simulink model "stream_mdbrt_backup5"  (R2023b)
settings: Solver=VariableStepAuto  StartTime=0.0  StopTime=(48)/fs  RelTol=1e-3
PreLoadFcn:
  | clear all;
  | 
  | fs = 100e6;
PostLoadFcn:
  | ratio = 1/6;
  | set(0,'units','pixels');
  | pixels = get(0,'screensize');
  | point1 = round(pixels(3)*ratio);
  | point2 = round(pixels(4)*ratio);
  | point3 = pixels(3)-round(pixels(3)*ratio);
  | point4 = pixels(4)-round(pixels(4)*ratio);
  | h = get_param(gcs,'handle');
  | set_param(h,'location',[point1 point2 point3 point4]);
  | pause(0.2);
  | set_param(h,'Zoomfactor','fit to view');
  | 
  | clear ratio pixels point1 point2 point3 point4 h
  | 
  | % https://uk.mathworks.com/matlabcentral/answers/358413-open-simulink-model-with-set-window-size-and-position
undefined symbols (not defined in the file): AXI4, bits, bitsheight, bitsiter, bitswidth, Lite, xc7z020clg400
libraries: hdlBasic x527, vmcUtilities x1
(part 3 of 5)

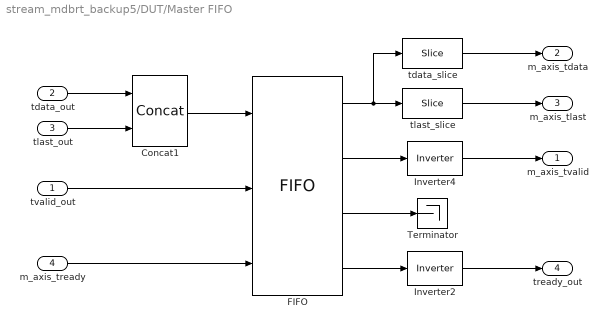
== system stream_mdbrt_backup5/DUT/Master FIFO ==
  tvalid_out : Inport
  tdata_out : Inport  Port=2
  tlast_out : Inport  Port=3
  m_axis_tready : Inport  Port=4
  Concat1 : hdlBasic/Concat  num_inputs=2  XmcBlockStatus=1  maskContainerNames=group1  block_type=concat  block_config=sysgen:Concat_config
  FIFO : hdlBasic/FIFO  mem_type=Block RAM  performance_options=First_Word_Fall_Through  embedded_registers=off  depth=1K  use_asym_data_widths=off  asym_read_width=32  percent_nbits=1  rst=off  rst_latency=1  en=off  use_dcount=off  use_percent_full_port=off  use_almost_empty=off  almost_empty_thresh=2  use_almost_full=on  use_rd_rst_busy=off  use_wr_rst_busy=off  almost_full_thresh=1000  almost_empty_offset=[]  almost_full_offset=[]  explicit_period=off  period=[]  store_only_valid=[]  init_zero=[]  simulation_type=fast_sim  XmcBlockStatus=1  maskContainerNames=tabcontainer1  block_type=fifo  block_config=sysgen:FIFO_config  block_width=538  block_height=997
      settings: infoedit=[]
  Inverter2 : hdlBasic/Inverter  en=off  latency=0  XmcBlockStatus=1  maskContainerNames=group2  block_type=inv  block_config=sysgen:Inverter_config
  Inverter4 : hdlBasic/Inverter  en=off  latency=0  XmcBlockStatus=1  maskContainerNames=group2  block_type=inv  block_config=sysgen:Inverter_config
  Terminator : Terminator
  tdata_slice : hdlBasic/Slice  nbits=1  boolean_output=off  mode=Two Bit Locations  bit1=0  base1=MSB of Input  bit0=1  base0=LSB of Input  XmcBlockStatus=1  maskContainerNames=group1  block_type=slice  block_config=sysgen:Slice_config
  tlast_slice : hdlBasic/Slice  nbits=1  boolean_output=on  mode=Two Bit Locations  bit1=0  base1=LSB of Input  bit0=0  base0=LSB of Input  XmcBlockStatus=1  maskContainerNames=group1  block_type=slice  block_config=sysgen:Slice_config
  m_axis_tvalid : Outport
  m_axis_tdata : Outport  Port=2
  m_axis_tlast : Outport  Port=3
  tready_out : Outport  Port=4
  wires:
  FIFO/4 -> Inverter2/1
  Inverter2/1 -> tready_out/1
  FIFO/2 -> Inverter4/1
  FIFO/1 -> tlast_slice/1, tdata_slice/1
  tlast_slice/1 -> m_axis_tlast/1
  tdata_slice/1 -> m_axis_tdata/1
  m_axis_tready/1 -> FIFO/3
  tvalid_out/1 -> FIFO/2
  Concat1/1 -> FIFO/1
  tdata_out/1 -> Concat1/1
  tlast_out/1 -> Concat1/2
  Inverter4/1 -> m_axis_tvalid/1
  FIFO/3 -> Terminator/1

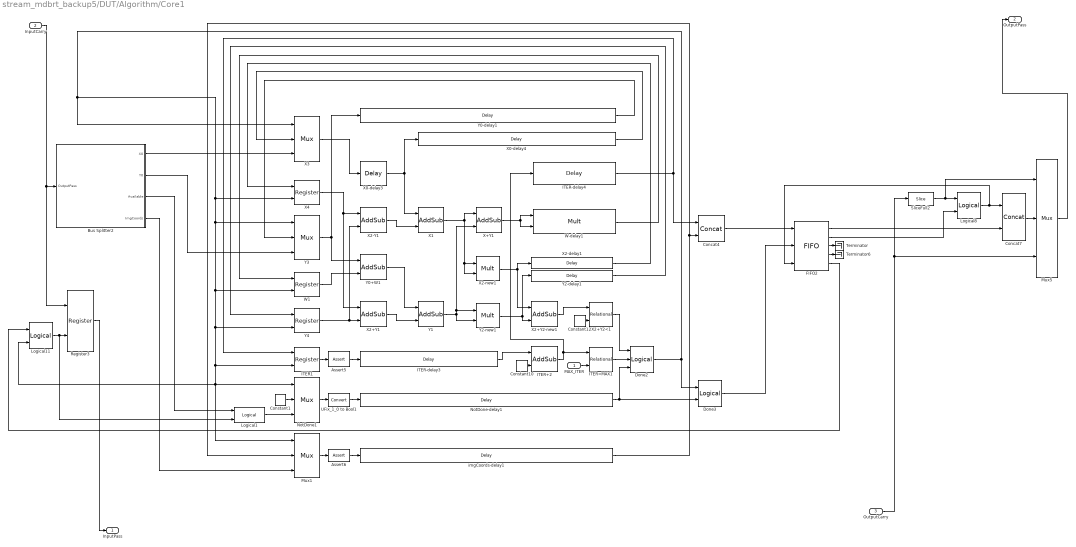
== system stream_mdbrt_backup5/DUT/Algorithm/Core1 ==
  MAX_ITER : Inport
  InputCarry : Inport  Port=2
  OutputCarry : Inport  Port=3
  Assert5 : hdlBasic/Assert  assert_type=on  type_source=Explicitly  gui_display_data_type=Fixed-point  arith_type=Unsigned  n_bits=bitsiter  bin_pt=0  preci_type=Single  exp_width=8  frac_width=24  assert_rate=off  rate_source=Explicitly  period=1  output_port=on  XmcBlockStatus=1  maskContainerNames=group1  block_type=assert  block_config=sysgen:assert_config  block_width=609  block_height=900
  Assert6 : hdlBasic/Assert  assert_type=on  type_source=Explicitly  gui_display_data_type=Fixed-point  arith_type=Unsigned  n_bits=bitswidth+bitsheight  bin_pt=0  preci_type=Single  exp_width=8  frac_width=24  assert_rate=off  rate_source=Explicitly  period=1  output_port=on  XmcBlockStatus=1  maskContainerNames=group1  block_type=assert  block_config=sysgen:assert_config  block_width=609  block_height=900
  Bus Splitter2 : Subsystem  TreatAsAtomicUnit=on
  Concat4 : hdlBasic/Concat  num_inputs=2  XmcBlockStatus=1  maskContainerNames=group1  block_type=concat  block_config=sysgen:Concat_config
  Concat7 : hdlBasic/Concat  num_inputs=2  XmcBlockStatus=1  maskContainerNames=group1  block_type=concat  block_config=sysgen:Concat_config
  Constant1 : hdlBasic/Constant  const=1  gui_display_data_type=Boolean  arith_type=Boolean  n_bits=bits  bin_pt=0  preci_type=Single  exp_width=8  frac_width=24  explicit_period=off  period=1  XmcBlockStatus=1  maskContainerNames=tabcontainer1  block_type=constant  block_config=sysgen:Constant_config
  Constant10 : hdlBasic/Constant  const=1  gui_display_data_type=Fixed-point  arith_type=Unsigned  n_bits=bits  bin_pt=0  preci_type=Single  exp_width=8  frac_width=24  explicit_period=off  period=1  XmcBlockStatus=1  maskContainerNames=tabcontainer1  block_type=constant  block_config=sysgen:Constant_config
  Constant12 : hdlBasic/Constant  const=4  gui_display_data_type=Fixed-point  arith_type=Signed (2's comp)  n_bits=bits  bin_pt=binpoint  preci_type=Single  exp_width=8  frac_width=24  explicit_period=off  period=1  XmcBlockStatus=1  maskContainerNames=tabcontainer1  block_type=constant  block_config=sysgen:Constant_config
  Done2 : hdlBasic/Logical  logical_function=NAND  inputs=3  en=off  latency=0  precision=User Defined  arith_type=Boolean  n_bits=1  bin_pt=0  align_bp=on  overflow=[]  quantization=[]  XmcBlockStatus=1  maskContainerNames=tabcontainer1  block_type=logical  block_config=sysgen:Logical_config
  Done3 : hdlBasic/Logical  logical_function=AND  inputs=2  en=off  latency=0  precision=User Defined  arith_type=Boolean  n_bits=1  bin_pt=0  align_bp=on  overflow=[]  quantization=[]  XmcBlockStatus=1  maskContainerNames=tabcontainer1  block_type=logical  block_config=sysgen:Logical_config
  FIFO2 : hdlBasic/FIFO  mem_type=Distributed RAM  performance_options=First_Word_Fall_Through  embedded_registers=off  depth=32  use_asym_data_widths=off  asym_read_width=32  percent_nbits=1  rst=off  rst_latency=1  en=off  use_dcount=off  use_percent_full_port=on  use_almost_empty=on  almost_empty_thresh=15  use_almost_full=off  use_rd_rst_busy=off  use_wr_rst_busy=off  almost_full_thresh=7  almost_empty_offset=[]  almost_full_offset=[]  explicit_period=off  period=[]  store_only_valid=[]  init_zero=[]  simulation_type=fast_sim  XmcBlockStatus=1  maskContainerNames=tabcontainer1  block_type=fifo  block_config=sysgen:FIFO_config  block_width=538  block_height=997
      settings: infoedit=[]
  ITER+2 : hdlBasic/AddSub  mode=Addition  use_carryin=off  use_carryout=off  en=off  latency=3  precision=User Defined  arith_type=Unsigned  n_bits=bitsiter  bin_pt=0  quantization=Truncate  overflow=Wrap  use_behavioral_HDL=off  hw_selection=Fabric  pipelined=off  XmcBlockStatus=1  maskContainerNames=tabcontainer1  block_type=addsub  block_config=sysgen:Addsub_config
  ITER-delay3 : hdlBasic/Delay  rst=off  en=off  latency=8  reg_retiming=off  XmcBlockStatus=1  maskContainerNames=group1  block_type=delay  block_config=sysgen:Delay_config
  ITER-delay4 : hdlBasic/Delay  rst=off  en=off  latency=2  reg_retiming=off  XmcBlockStatus=1  maskContainerNames=group1  block_type=delay  block_config=sysgen:Delay_config
  ITER1 : hdlBasic/Register  init=0  rst=on  en=off  XmcBlockStatus=1  maskContainerNames=tabcontainer1  block_type=register  block_config=sysgen:Register_config
  ITER<MAX1 : hdlBasic/Relational  mode=a<b  op_type=Bool  en=off  latency=2  XmcBlockStatus=1  maskContainerNames=tabcontainer1  block_type=relational  block_config=sysgen:Relational_config
  Logical1 : hdlBasic/Logical  logical_function=AND  inputs=2  en=off  latency=0  precision=Full  arith_type=Unsigned  n_bits=16  bin_pt=0  align_bp=on  overflow=[]  quantization=[]  XmcBlockStatus=1  maskContainerNames=tabcontainer1  block_type=logical  block_config=sysgen:Logical_config
  Logical11 : hdlBasic/Logical  logical_function=AND  inputs=2  en=off  latency=0  precision=Full  arith_type=Unsigned  n_bits=16  bin_pt=0  align_bp=on  overflow=[]  quantization=[]  XmcBlockStatus=1  maskContainerNames=tabcontainer1  block_type=logical  block_config=sysgen:Logical_config
  Logical8 : hdlBasic/Logical  logical_function=NOR  inputs=2  en=off  latency=0  precision=Full  arith_type=Unsigned  n_bits=16  bin_pt=0  align_bp=on  overflow=[]  quantization=[]  XmcBlockStatus=1  maskContainerNames=tabcontainer1  block_type=logical  block_config=sysgen:Logical_config
  Mux1 : hdlBasic/Mux  inputs=2  en=off  latency=1  precision=User Defined  arith_type=Unsigned  n_bits=bitswidth+bitsheight  bin_pt=0  quantization=Truncate  overflow=Wrap  XmcBlockStatus=1  maskContainerNames=tabcontainer1  block_type=mux  block_config=sysgen:Mux_config
  Mux5 : hdlBasic/Mux  inputs=2  en=off  latency=1  precision=User Defined  arith_type=Unsigned  n_bits=bitswidth+bitsheight+bitsiter+1  bin_pt=0  quantization=Truncate  overflow=Wrap  XmcBlockStatus=1  maskContainerNames=tabcontainer1  block_type=mux  block_config=sysgen:Mux_config
  NotDone-delay1 : hdlBasic/Delay  rst=off  en=off  latency=13  reg_retiming=off  XmcBlockStatus=1  maskContainerNames=group1  block_type=delay  block_config=sysgen:Delay_config
  NotDone1 : hdlBasic/Mux  inputs=2  en=off  latency=1  precision=User Defined  arith_type=Unsigned  n_bits=1  bin_pt=0  quantization=Truncate  overflow=Wrap  XmcBlockStatus=1  maskContainerNames=tabcontainer1  block_type=mux  block_config=sysgen:Mux_config
  Register3 : hdlBasic/Register  init=0  rst=on  en=off  XmcBlockStatus=1  maskContainerNames=tabcontainer1  block_type=register  block_config=sysgen:Register_config
  SliceFull2 : hdlBasic/Slice  nbits=1  boolean_output=on  mode=Upper Bit Location + Width  bit1=0  base1=MSB of Input  bit0=0  base0=LSB of Input  XmcBlockStatus=1  maskContainerNames=group1  block_type=slice  block_config=sysgen:Slice_config
  Terminator : Terminator
  Terminator6 : Terminator
  UFix_1_0 to Bool1 : hdlBasic/Convert  gui_display_data_type=Boolean  arith_type=Boolean  n_bits=16  bin_pt=14  float_type=Single  exp_bits=8  fraction_bits=24  quantization=Truncate  overflow=Wrap  en=off  latency=0  pipeline=off  XmcBlockStatus=1  maskContainerNames=group2  block_type=convert  block_config=sysgen:Convert_config  block_width=595  block_height=885
  W-delay1 : hdlBasic/Mult  precision=Full  arith_type="Signed  (2's comp)"  n_bits=16  bin_pt=14  quantization=Truncate  overflow=Wrap  en=off  latency=7  use_behavioral_HDL=off  opt=Speed  use_embedded=on  optimum_pipeline=off  pipeline=on  use_rpm=on  placement_style=Triangular  XmcBlockStatus=1  maskContainerNames=group1  block_type=mult  block_config=sysgen:Mult_config  block_width=598  block_height=876
  W1 : hdlBasic/Register  init=0  rst=on  en=off  XmcBlockStatus=1  maskContainerNames=tabcontainer1  block_type=register  block_config=sysgen:Register_config
  X+Y1 : hdlBasic/AddSub  mode=Addition  use_carryin=off  use_carryout=off  en=off  latency=4  precision=User Defined  arith_type="Signed  (2's comp)"  n_bits=bits  bin_pt=binpoint  quantization=Truncate  overflow=Wrap  use_behavioral_HDL=off  hw_selection=Fabric  pipelined=off  XmcBlockStatus=1  maskContainerNames=tabcontainer1  block_type=addsub  block_config=sysgen:Addsub_config
  X0-delay3 : hdlBasic/Delay  rst=off  en=off  latency=1  reg_retiming=off  XmcBlockStatus=1  maskContainerNames=group1  block_type=delay  block_config=sysgen:Delay_config
  X0-delay4 : hdlBasic/Delay  rst=off  en=off  latency=12  reg_retiming=off  XmcBlockStatus=1  maskContainerNames=group1  block_type=delay  block_config=sysgen:Delay_config
  X1 : hdlBasic/AddSub  mode=Addition  use_carryin=off  use_carryout=off  en=off  latency=1  precision=User Defined  arith_type="Signed  (2's comp)"  n_bits=bits  bin_pt=binpoint  quantization=Truncate  overflow=Wrap  use_behavioral_HDL=off  hw_selection=Fabric  pipelined=off  XmcBlockStatus=1  maskContainerNames=tabcontainer1  block_type=addsub  block_config=sysgen:Addsub_config
  X2+Y1 : hdlBasic/AddSub  mode=Addition  use_carryin=off  use_carryout=off  en=off  latency=1  precision=User Defined  arith_type="Signed  (2's comp)"  n_bits=bits  bin_pt=binpoint  quantization=Truncate  overflow=Wrap  use_behavioral_HDL=off  hw_selection=Fabric  pipelined=off  XmcBlockStatus=1  maskContainerNames=tabcontainer1  block_type=addsub  block_config=sysgen:Addsub_config
  X2+Y2-new1 : hdlBasic/AddSub  mode=Addition  use_carryin=off  use_carryout=off  en=off  latency=3  precision=User Defined  arith_type="Signed  (2's comp)"  n_bits=bits  bin_pt=binpoint  quantization=Truncate  overflow=Wrap  use_behavioral_HDL=off  hw_selection=Fabric  pipelined=off  XmcBlockStatus=1  maskContainerNames=tabcontainer1  block_type=addsub  block_config=sysgen:Addsub_config
  X2+Y2<1 : hdlBasic/Relational  mode=a<b  op_type=Bool  en=off  latency=2  XmcBlockStatus=1  maskContainerNames=tabcontainer1  block_type=relational  block_config=sysgen:Relational_config
  X2-Y1 : hdlBasic/AddSub  mode=Subtraction  use_carryin=off  use_carryout=off  en=off  latency=1  precision=User Defined  arith_type="Signed  (2's comp)"  n_bits=bits  bin_pt=binpoint  quantization=Truncate  overflow=Wrap  use_behavioral_HDL=off  hw_selection=Fabric  pipelined=off  XmcBlockStatus=1  maskContainerNames=tabcontainer1  block_type=addsub  block_config=sysgen:Addsub_config
  X2-delay1 : hdlBasic/Delay  rst=off  en=off  latency=5  reg_retiming=off  XmcBlockStatus=1  maskContainerNames=group1  block_type=delay  block_config=sysgen:Delay_config
  X2-new1 : hdlBasic/Mult  precision=Full  arith_type="Signed  (2's comp)"  n_bits=16  bin_pt=14  quantization=Truncate  overflow=Wrap  en=off  latency=6  use_behavioral_HDL=off  opt=Speed  use_embedded=on  optimum_pipeline=off  pipeline=on  use_rpm=on  placement_style=Triangular  XmcBlockStatus=1  maskContainerNames=group1  block_type=mult  block_config=sysgen:Mult_config  block_width=598  block_height=876
  X3 : hdlBasic/Mux  inputs=2  en=off  latency=1  precision=User Defined  arith_type="Signed  (2's comp)"  n_bits=bits  bin_pt=binpoint  quantization=Truncate  overflow=Wrap  XmcBlockStatus=1  maskContainerNames=tabcontainer1  block_type=mux  block_config=sysgen:Mux_config
  X4 : hdlBasic/Register  init=0  rst=on  en=off  XmcBlockStatus=1  maskContainerNames=tabcontainer1  block_type=register  block_config=sysgen:Register_config
  Y0+W1 : hdlBasic/AddSub  mode=Addition  use_carryin=off  use_carryout=off  en=off  latency=1  precision=User Defined  arith_type="Signed  (2's comp)"  n_bits=bits  bin_pt=binpoint  quantization=Truncate  overflow=Wrap  use_behavioral_HDL=off  hw_selection=Fabric  pipelined=off  XmcBlockStatus=1  maskContainerNames=tabcontainer1  block_type=addsub  block_config=sysgen:Addsub_config
  Y0-delay1 : hdlBasic/Delay  rst=off  en=off  latency=13  reg_retiming=off  XmcBlockStatus=1  maskContainerNames=group1  block_type=delay  block_config=sysgen:Delay_config
  Y1 : hdlBasic/AddSub  mode=Subtraction  use_carryin=off  use_carryout=off  en=off  latency=1  precision=User Defined  arith_type="Signed  (2's comp)"  n_bits=bits  bin_pt=binpoint  quantization=Truncate  overflow=Wrap  use_behavioral_HDL=off  hw_selection=Fabric  pipelined=off  XmcBlockStatus=1  maskContainerNames=tabcontainer1  block_type=addsub  block_config=sysgen:Addsub_config
  Y2-delay1 : hdlBasic/Delay  rst=off  en=off  latency=5  reg_retiming=off  XmcBlockStatus=1  maskContainerNames=group1  block_type=delay  block_config=sysgen:Delay_config
  Y2-new1 : hdlBasic/Mult  precision=Full  arith_type="Signed  (2's comp)"  n_bits=16  bin_pt=14  quantization=Truncate  overflow=Wrap  en=off  latency=6  use_behavioral_HDL=off  opt=Speed  use_embedded=on  optimum_pipeline=off  pipeline=on  use_rpm=on  placement_style=Triangular  XmcBlockStatus=1  maskContainerNames=group1  block_type=mult  block_config=sysgen:Mult_config  block_width=598  block_height=876
  Y3 : hdlBasic/Mux  inputs=2  en=off  latency=1  precision=User Defined  arith_type="Signed  (2's comp)"  n_bits=bits  bin_pt=binpoint  quantization=Truncate  overflow=Wrap  XmcBlockStatus=1  maskContainerNames=tabcontainer1  block_type=mux  block_config=sysgen:Mux_config
  Y4 : hdlBasic/Register  init=0  rst=on  en=off  XmcBlockStatus=1  maskContainerNames=tabcontainer1  block_type=register  block_config=sysgen:Register_config
  imgCoords-delay1 : hdlBasic/Delay  rst=off  en=off  latency=13  reg_retiming=off  XmcBlockStatus=1  maskContainerNames=group1  block_type=delay  block_config=sysgen:Delay_config
  InputPass : Outport
  OutputPass : Outport  Port=2
  wires:
  NotDone1/1 -> UFix_1_0 to Bool1/1
  SliceFull2/1 -> Mux5/1, Logical8/1
  ITER-delay3/1 -> ITER+2/1
  Y4/1 -> X2-Y1/2, X2+Y1/2
  Y2-delay1/1 -> Y4/1
  Done3/1 -> FIFO2/2
  Assert6/1 -> imgCoords-delay1/1
  InputCarry/1 -> Register3/1, Bus Splitter2/1(OutputPass)
  X1/1 -> X2-new1/2, X2-new1/1, X+Y1/1
  X2-delay1/1 -> X4/1
  Done2/1 -> Done3/1, X4/2, Y3/1, W1/2, ITER1/2, Logical11/2, Mux1/1, NotDone1/1, Y4/2, X3/1
  W1/1 -> Y0+W1/2
  Constant10/1 -> ITER+2/2
  Logical8/1 -> FIFO2/3, Concat7/1
  FIFO2/2 -> Logical8/2
  X2+Y2-new1/1 -> X2+Y2<1/1
  Bus Splitter2/1(X0) -> X3/3
  X2+Y1/1 -> Y1/2
  Logical11/1 -> Logical1/2, Register3/2
  NotDone-delay1/1 -> Done2/3, Done3/2
  OutputCarry/1 -> SliceFull2/1, Mux5/3
  Mux5/1 -> OutputPass/1
  FIFO2/3 -> Terminator/1
  ITER-delay4/1 -> Concat4/1, ITER1/1
  Y3/1 -> Y0+W1/1, Y0-delay1/1
  Register3/1 -> InputPass/1
  X4/1 -> X2+Y1/1, X2-Y1/1
  ITER+2/1 -> ITER-delay4/1, ITER<MAX1/1
  Y1/1 -> X+Y1/2, Y2-new1/1, Y2-new1/2
  Y2-new1/1 -> Y2-delay1/1, X2+Y2-new1/2
  ITER<MAX1/1 -> Done2/2
  Constant12/1 -> X2+Y2<1/2
  Y0+W1/1 -> Y1/1
  Assert5/1 -> ITER-delay3/1
  UFix_1_0 to Bool1/1 -> NotDone-delay1/1
  X2+Y2<1/1 -> Done2/1
  imgCoords-delay1/1 -> Mux1/2, Concat4/2
  FIFO2/5 -> Logical11/1
  Bus Splitter2/4(ImgCoords) -> Mux1/3
  X2-Y1/1 -> X1/2
  ITER1/1 -> Assert5/1
  X+Y1/1 -> W-delay1/2, W-delay1/1
  X0-delay3/1 -> X0-delay4/1, X1/1
  Y0-delay1/1 -> Y3/2
  X3/1 -> X0-delay3/1
  Concat7/1 -> Mux5/2
  X0-delay4/1 -> X3/2
  X2-new1/1 -> X2-delay1/1, X2+Y2-new1/1
  Bus Splitter2/2(Y0) -> Y3/3
  W-delay1/1 -> W1/1
  MAX_ITER/1 -> ITER<MAX1/2
  Bus Splitter2/3(Available) -> Logical1/1
  FIFO2/4 -> Terminator6/1
  Mux1/1 -> Assert6/1
  Concat4/1 -> FIFO2/1
  FIFO2/1 -> Concat7/2
  Constant1/1 -> NotDone1/2
  Logical1/1 -> NotDone1/3

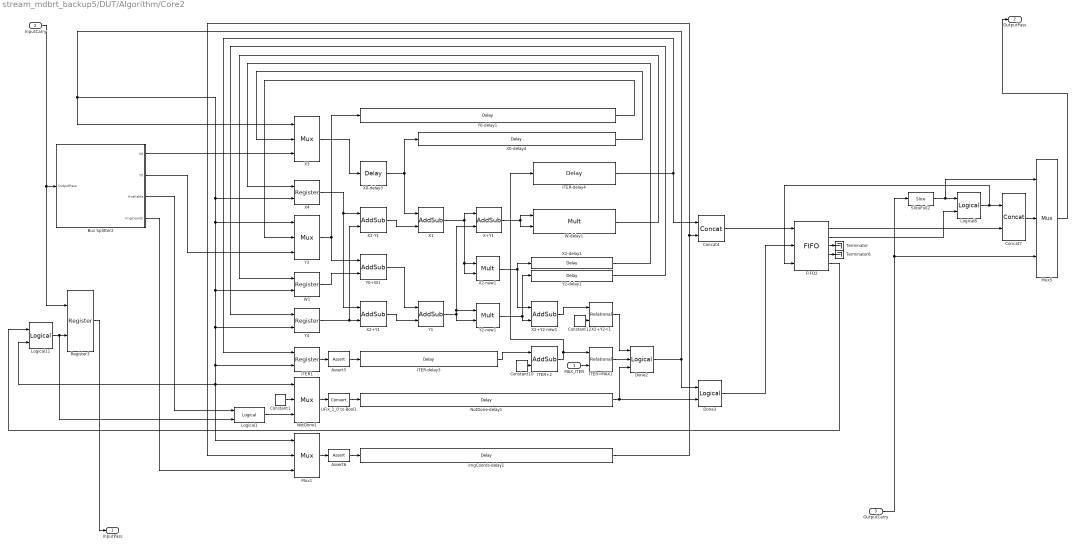
== system stream_mdbrt_backup5/DUT/Algorithm/Core2 ==
  MAX_ITER : Inport
  InputCarry : Inport  Port=2
  OutputCarry : Inport  Port=3
  Assert5 : hdlBasic/Assert  assert_type=on  type_source=Explicitly  gui_display_data_type=Fixed-point  arith_type=Unsigned  n_bits=bitsiter  bin_pt=0  preci_type=Single  exp_width=8  frac_width=24  assert_rate=off  rate_source=Explicitly  period=1  output_port=on  XmcBlockStatus=1  maskContainerNames=group1  block_type=assert  block_config=sysgen:assert_config  block_width=609  block_height=900
  Assert6 : hdlBasic/Assert  assert_type=on  type_source=Explicitly  gui_display_data_type=Fixed-point  arith_type=Unsigned  n_bits=bitswidth+bitsheight  bin_pt=0  preci_type=Single  exp_width=8  frac_width=24  assert_rate=off  rate_source=Explicitly  period=1  output_port=on  XmcBlockStatus=1  maskContainerNames=group1  block_type=assert  block_config=sysgen:assert_config  block_width=609  block_height=900
  Bus Splitter2 : Subsystem  TreatAsAtomicUnit=on
  Concat4 : hdlBasic/Concat  num_inputs=2  XmcBlockStatus=1  maskContainerNames=group1  block_type=concat  block_config=sysgen:Concat_config
  Concat7 : hdlBasic/Concat  num_inputs=2  XmcBlockStatus=1  maskContainerNames=group1  block_type=concat  block_config=sysgen:Concat_config
  Constant1 : hdlBasic/Constant  const=1  gui_display_data_type=Boolean  arith_type=Boolean  n_bits=bits  bin_pt=0  preci_type=Single  exp_width=8  frac_width=24  explicit_period=off  period=1  XmcBlockStatus=1  maskContainerNames=tabcontainer1  block_type=constant  block_config=sysgen:Constant_config
  Constant10 : hdlBasic/Constant  const=1  gui_display_data_type=Fixed-point  arith_type=Unsigned  n_bits=bits  bin_pt=0  preci_type=Single  exp_width=8  frac_width=24  explicit_period=off  period=1  XmcBlockStatus=1  maskContainerNames=tabcontainer1  block_type=constant  block_config=sysgen:Constant_config
  Constant12 : hdlBasic/Constant  const=4  gui_display_data_type=Fixed-point  arith_type=Signed (2's comp)  n_bits=bits  bin_pt=binpoint  preci_type=Single  exp_width=8  frac_width=24  explicit_period=off  period=1  XmcBlockStatus=1  maskContainerNames=tabcontainer1  block_type=constant  block_config=sysgen:Constant_config
  Done2 : hdlBasic/Logical  logical_function=NAND  inputs=3  en=off  latency=0  precision=User Defined  arith_type=Boolean  n_bits=1  bin_pt=0  align_bp=on  overflow=[]  quantization=[]  XmcBlockStatus=1  maskContainerNames=tabcontainer1  block_type=logical  block_config=sysgen:Logical_config
  Done3 : hdlBasic/Logical  logical_function=AND  inputs=2  en=off  latency=0  precision=User Defined  arith_type=Boolean  n_bits=1  bin_pt=0  align_bp=on  overflow=[]  quantization=[]  XmcBlockStatus=1  maskContainerNames=tabcontainer1  block_type=logical  block_config=sysgen:Logical_config
  FIFO2 : hdlBasic/FIFO  mem_type=Distributed RAM  performance_options=First_Word_Fall_Through  embedded_registers=off  depth=32  use_asym_data_widths=off  asym_read_width=32  percent_nbits=1  rst=off  rst_latency=1  en=off  use_dcount=off  use_percent_full_port=on  use_almost_empty=on  almost_empty_thresh=15  use_almost_full=off  use_rd_rst_busy=off  use_wr_rst_busy=off  almost_full_thresh=7  almost_empty_offset=[]  almost_full_offset=[]  explicit_period=off  period=[]  store_only_valid=[]  init_zero=[]  simulation_type=fast_sim  XmcBlockStatus=1  maskContainerNames=tabcontainer1  block_type=fifo  block_config=sysgen:FIFO_config  block_width=538  block_height=997
      settings: infoedit=[]
  ITER+2 : hdlBasic/AddSub  mode=Addition  use_carryin=off  use_carryout=off  en=off  latency=3  precision=User Defined  arith_type=Unsigned  n_bits=bitsiter  bin_pt=0  quantization=Truncate  overflow=Wrap  use_behavioral_HDL=off  hw_selection=Fabric  pipelined=off  XmcBlockStatus=1  maskContainerNames=tabcontainer1  block_type=addsub  block_config=sysgen:Addsub_config
  ITER-delay3 : hdlBasic/Delay  rst=off  en=off  latency=8  reg_retiming=off  XmcBlockStatus=1  maskContainerNames=group1  block_type=delay  block_config=sysgen:Delay_config
  ITER-delay4 : hdlBasic/Delay  rst=off  en=off  latency=2  reg_retiming=off  XmcBlockStatus=1  maskContainerNames=group1  block_type=delay  block_config=sysgen:Delay_config
  ITER1 : hdlBasic/Register  init=0  rst=on  en=off  XmcBlockStatus=1  maskContainerNames=tabcontainer1  block_type=register  block_config=sysgen:Register_config
  ITER<MAX1 : hdlBasic/Relational  mode=a<b  op_type=Bool  en=off  latency=2  XmcBlockStatus=1  maskContainerNames=tabcontainer1  block_type=relational  block_config=sysgen:Relational_config
  Logical1 : hdlBasic/Logical  logical_function=AND  inputs=2  en=off  latency=0  precision=Full  arith_type=Unsigned  n_bits=16  bin_pt=0  align_bp=on  overflow=[]  quantization=[]  XmcBlockStatus=1  maskContainerNames=tabcontainer1  block_type=logical  block_config=sysgen:Logical_config
  Logical11 : hdlBasic/Logical  logical_function=AND  inputs=2  en=off  latency=0  precision=Full  arith_type=Unsigned  n_bits=16  bin_pt=0  align_bp=on  overflow=[]  quantization=[]  XmcBlockStatus=1  maskContainerNames=tabcontainer1  block_type=logical  block_config=sysgen:Logical_config
  Logical8 : hdlBasic/Logical  logical_function=NOR  inputs=2  en=off  latency=0  precision=Full  arith_type=Unsigned  n_bits=16  bin_pt=0  align_bp=on  overflow=[]  quantization=[]  XmcBlockStatus=1  maskContainerNames=tabcontainer1  block_type=logical  block_config=sysgen:Logical_config
  Mux1 : hdlBasic/Mux  inputs=2  en=off  latency=1  precision=User Defined  arith_type=Unsigned  n_bits=bitswidth+bitsheight  bin_pt=0  quantization=Truncate  overflow=Wrap  XmcBlockStatus=1  maskContainerNames=tabcontainer1  block_type=mux  block_config=sysgen:Mux_config
  Mux5 : hdlBasic/Mux  inputs=2  en=off  latency=1  precision=User Defined  arith_type=Unsigned  n_bits=bitswidth+bitsheight+bitsiter+1  bin_pt=0  quantization=Truncate  overflow=Wrap  XmcBlockStatus=1  maskContainerNames=tabcontainer1  block_type=mux  block_config=sysgen:Mux_config
  NotDone-delay1 : hdlBasic/Delay  rst=off  en=off  latency=13  reg_retiming=off  XmcBlockStatus=1  maskContainerNames=group1  block_type=delay  block_config=sysgen:Delay_config
  NotDone1 : hdlBasic/Mux  inputs=2  en=off  latency=1  precision=User Defined  arith_type=Unsigned  n_bits=1  bin_pt=0  quantization=Truncate  overflow=Wrap  XmcBlockStatus=1  maskContainerNames=tabcontainer1  block_type=mux  block_config=sysgen:Mux_config
  Register3 : hdlBasic/Register  init=0  rst=on  en=off  XmcBlockStatus=1  maskContainerNames=tabcontainer1  block_type=register  block_config=sysgen:Register_config
  SliceFull2 : hdlBasic/Slice  nbits=1  boolean_output=on  mode=Upper Bit Location + Width  bit1=0  base1=MSB of Input  bit0=0  base0=LSB of Input  XmcBlockStatus=1  maskContainerNames=group1  block_type=slice  block_config=sysgen:Slice_config
  Terminator : Terminator
  Terminator6 : Terminator
  UFix_1_0 to Bool1 : hdlBasic/Convert  gui_display_data_type=Boolean  arith_type=Boolean  n_bits=16  bin_pt=14  float_type=Single  exp_bits=8  fraction_bits=24  quantization=Truncate  overflow=Wrap  en=off  latency=0  pipeline=off  XmcBlockStatus=1  maskContainerNames=group2  block_type=convert  block_config=sysgen:Convert_config  block_width=595  block_height=885
  W-delay1 : hdlBasic/Mult  precision=Full  arith_type="Signed  (2's comp)"  n_bits=16  bin_pt=14  quantization=Truncate  overflow=Wrap  en=off  latency=7  use_behavioral_HDL=off  opt=Speed  use_embedded=on  optimum_pipeline=off  pipeline=on  use_rpm=on  placement_style=Triangular  XmcBlockStatus=1  maskContainerNames=group1  block_type=mult  block_config=sysgen:Mult_config  block_width=598  block_height=876
  W1 : hdlBasic/Register  init=0  rst=on  en=off  XmcBlockStatus=1  maskContainerNames=tabcontainer1  block_type=register  block_config=sysgen:Register_config
  X+Y1 : hdlBasic/AddSub  mode=Addition  use_carryin=off  use_carryout=off  en=off  latency=4  precision=User Defined  arith_type="Signed  (2's comp)"  n_bits=bits  bin_pt=binpoint  quantization=Truncate  overflow=Wrap  use_behavioral_HDL=off  hw_selection=Fabric  pipelined=off  XmcBlockStatus=1  maskContainerNames=tabcontainer1  block_type=addsub  block_config=sysgen:Addsub_config
  X0-delay3 : hdlBasic/Delay  rst=off  en=off  latency=1  reg_retiming=off  XmcBlockStatus=1  maskContainerNames=group1  block_type=delay  block_config=sysgen:Delay_config
  X0-delay4 : hdlBasic/Delay  rst=off  en=off  latency=12  reg_retiming=off  XmcBlockStatus=1  maskContainerNames=group1  block_type=delay  block_config=sysgen:Delay_config
  X1 : hdlBasic/AddSub  mode=Addition  use_carryin=off  use_carryout=off  en=off  latency=1  precision=User Defined  arith_type="Signed  (2's comp)"  n_bits=bits  bin_pt=binpoint  quantization=Truncate  overflow=Wrap  use_behavioral_HDL=off  hw_selection=Fabric  pipelined=off  XmcBlockStatus=1  maskContainerNames=tabcontainer1  block_type=addsub  block_config=sysgen:Addsub_config
  X2+Y1 : hdlBasic/AddSub  mode=Addition  use_carryin=off  use_carryout=off  en=off  latency=1  precision=User Defined  arith_type="Signed  (2's comp)"  n_bits=bits  bin_pt=binpoint  quantization=Truncate  overflow=Wrap  use_behavioral_HDL=off  hw_selection=Fabric  pipelined=off  XmcBlockStatus=1  maskContainerNames=tabcontainer1  block_type=addsub  block_config=sysgen:Addsub_config
  X2+Y2-new1 : hdlBasic/AddSub  mode=Addition  use_carryin=off  use_carryout=off  en=off  latency=3  precision=User Defined  arith_type="Signed  (2's comp)"  n_bits=bits  bin_pt=binpoint  quantization=Truncate  overflow=Wrap  use_behavioral_HDL=off  hw_selection=Fabric  pipelined=off  XmcBlockStatus=1  maskContainerNames=tabcontainer1  block_type=addsub  block_config=sysgen:Addsub_config
  X2+Y2<1 : hdlBasic/Relational  mode=a<b  op_type=Bool  en=off  latency=2  XmcBlockStatus=1  maskContainerNames=tabcontainer1  block_type=relational  block_config=sysgen:Relational_config
  X2-Y1 : hdlBasic/AddSub  mode=Subtraction  use_carryin=off  use_carryout=off  en=off  latency=1  precision=User Defined  arith_type="Signed  (2's comp)"  n_bits=bits  bin_pt=binpoint  quantization=Truncate  overflow=Wrap  use_behavioral_HDL=off  hw_selection=Fabric  pipelined=off  XmcBlockStatus=1  maskContainerNames=tabcontainer1  block_type=addsub  block_config=sysgen:Addsub_config
  X2-delay1 : hdlBasic/Delay  rst=off  en=off  latency=5  reg_retiming=off  XmcBlockStatus=1  maskContainerNames=group1  block_type=delay  block_config=sysgen:Delay_config
  X2-new1 : hdlBasic/Mult  precision=Full  arith_type="Signed  (2's comp)"  n_bits=16  bin_pt=14  quantization=Truncate  overflow=Wrap  en=off  latency=6  use_behavioral_HDL=off  opt=Speed  use_embedded=on  optimum_pipeline=off  pipeline=on  use_rpm=on  placement_style=Triangular  XmcBlockStatus=1  maskContainerNames=group1  block_type=mult  block_config=sysgen:Mult_config  block_width=598  block_height=876
  X3 : hdlBasic/Mux  inputs=2  en=off  latency=1  precision=User Defined  arith_type="Signed  (2's comp)"  n_bits=bits  bin_pt=binpoint  quantization=Truncate  overflow=Wrap  XmcBlockStatus=1  maskContainerNames=tabcontainer1  block_type=mux  block_config=sysgen:Mux_config
  X4 : hdlBasic/Register  init=0  rst=on  en=off  XmcBlockStatus=1  maskContainerNames=tabcontainer1  block_type=register  block_config=sysgen:Register_config
  Y0+W1 : hdlBasic/AddSub  mode=Addition  use_carryin=off  use_carryout=off  en=off  latency=1  precision=User Defined  arith_type="Signed  (2's comp)"  n_bits=bits  bin_pt=binpoint  quantization=Truncate  overflow=Wrap  use_behavioral_HDL=off  hw_selection=Fabric  pipelined=off  XmcBlockStatus=1  maskContainerNames=tabcontainer1  block_type=addsub  block_config=sysgen:Addsub_config
  Y0-delay1 : hdlBasic/Delay  rst=off  en=off  latency=13  reg_retiming=off  XmcBlockStatus=1  maskContainerNames=group1  block_type=delay  block_config=sysgen:Delay_config
  Y1 : hdlBasic/AddSub  mode=Subtraction  use_carryin=off  use_carryout=off  en=off  latency=1  precision=User Defined  arith_type="Signed  (2's comp)"  n_bits=bits  bin_pt=binpoint  quantization=Truncate  overflow=Wrap  use_behavioral_HDL=off  hw_selection=Fabric  pipelined=off  XmcBlockStatus=1  maskContainerNames=tabcontainer1  block_type=addsub  block_config=sysgen:Addsub_config
  Y2-delay1 : hdlBasic/Delay  rst=off  en=off  latency=5  reg_retiming=off  XmcBlockStatus=1  maskContainerNames=group1  block_type=delay  block_config=sysgen:Delay_config
  Y2-new1 : hdlBasic/Mult  precision=Full  arith_type="Signed  (2's comp)"  n_bits=16  bin_pt=14  quantization=Truncate  overflow=Wrap  en=off  latency=6  use_behavioral_HDL=off  opt=Speed  use_embedded=on  optimum_pipeline=off  pipeline=on  use_rpm=on  placement_style=Triangular  XmcBlockStatus=1  maskContainerNames=group1  block_type=mult  block_config=sysgen:Mult_config  block_width=598  block_height=876
  Y3 : hdlBasic/Mux  inputs=2  en=off  latency=1  precision=User Defined  arith_type="Signed  (2's comp)"  n_bits=bits  bin_pt=binpoint  quantization=Truncate  overflow=Wrap  XmcBlockStatus=1  maskContainerNames=tabcontainer1  block_type=mux  block_config=sysgen:Mux_config
  Y4 : hdlBasic/Register  init=0  rst=on  en=off  XmcBlockStatus=1  maskContainerNames=tabcontainer1  block_type=register  block_config=sysgen:Register_config
  imgCoords-delay1 : hdlBasic/Delay  rst=off  en=off  latency=13  reg_retiming=off  XmcBlockStatus=1  maskContainerNames=group1  block_type=delay  block_config=sysgen:Delay_config
  InputPass : Outport
  OutputPass : Outport  Port=2
  wires:
  Logical1/1 -> NotDone1/3
  Constant1/1 -> NotDone1/2
  FIFO2/1 -> Concat7/2
  Concat4/1 -> FIFO2/1
  Mux1/1 -> Assert6/1
  FIFO2/4 -> Terminator6/1
  Bus Splitter2/3(Available) -> Logical1/1
  MAX_ITER/1 -> ITER<MAX1/2
  W-delay1/1 -> W1/1
  Bus Splitter2/2(Y0) -> Y3/3
  X2-new1/1 -> X2+Y2-new1/1, X2-delay1/1
  X0-delay4/1 -> X3/2
  Concat7/1 -> Mux5/2
  X3/1 -> X0-delay3/1
  Y0-delay1/1 -> Y3/2
  X0-delay3/1 -> X1/1, X0-delay4/1
  X+Y1/1 -> W-delay1/1, W-delay1/2
  ITER1/1 -> Assert5/1
  X2-Y1/1 -> X1/2
  Bus Splitter2/4(ImgCoords) -> Mux1/3
  FIFO2/5 -> Logical11/1
  imgCoords-delay1/1 -> Concat4/2, Mux1/2
  X2+Y2<1/1 -> Done2/1
  UFix_1_0 to Bool1/1 -> NotDone-delay1/1
  Assert5/1 -> ITER-delay3/1
  Y0+W1/1 -> Y1/1
  Constant12/1 -> X2+Y2<1/2
  ITER<MAX1/1 -> Done2/2
  Y2-new1/1 -> X2+Y2-new1/2, Y2-delay1/1
  Y1/1 -> Y2-new1/2, Y2-new1/1, X+Y1/2
  ITER+2/1 -> ITER<MAX1/1, ITER-delay4/1
  X4/1 -> X2-Y1/1, X2+Y1/1
  Register3/1 -> InputPass/1
  Y3/1 -> Y0-delay1/1, Y0+W1/1
  ITER-delay4/1 -> ITER1/1, Concat4/1
  FIFO2/3 -> Terminator/1
  Mux5/1 -> OutputPass/1
  OutputCarry/1 -> Mux5/3, SliceFull2/1
  NotDone-delay1/1 -> Done3/2, Done2/3
  Logical11/1 -> Register3/2, Logical1/2
  X2+Y1/1 -> Y1/2
  Bus Splitter2/1(X0) -> X3/3
  X2+Y2-new1/1 -> X2+Y2<1/1
  FIFO2/2 -> Logical8/2
  Logical8/1 -> Concat7/1, FIFO2/3
  Constant10/1 -> ITER+2/2
  W1/1 -> Y0+W1/2
  Done2/1 -> X3/1, Y4/2, NotDone1/1, Mux1/1, Logical11/2, ITER1/2, W1/2, Y3/1, X4/2, Done3/1
  X2-delay1/1 -> X4/1
  X1/1 -> X+Y1/1, X2-new1/1, X2-new1/2
  InputCarry/1 -> Bus Splitter2/1(OutputPass), Register3/1
  Assert6/1 -> imgCoords-delay1/1
  Done3/1 -> FIFO2/2
  Y2-delay1/1 -> Y4/1
  Y4/1 -> X2+Y1/2, X2-Y1/2
  ITER-delay3/1 -> ITER+2/1
  SliceFull2/1 -> Logical8/1, Mux5/1
  NotDone1/1 -> UFix_1_0 to Bool1/1

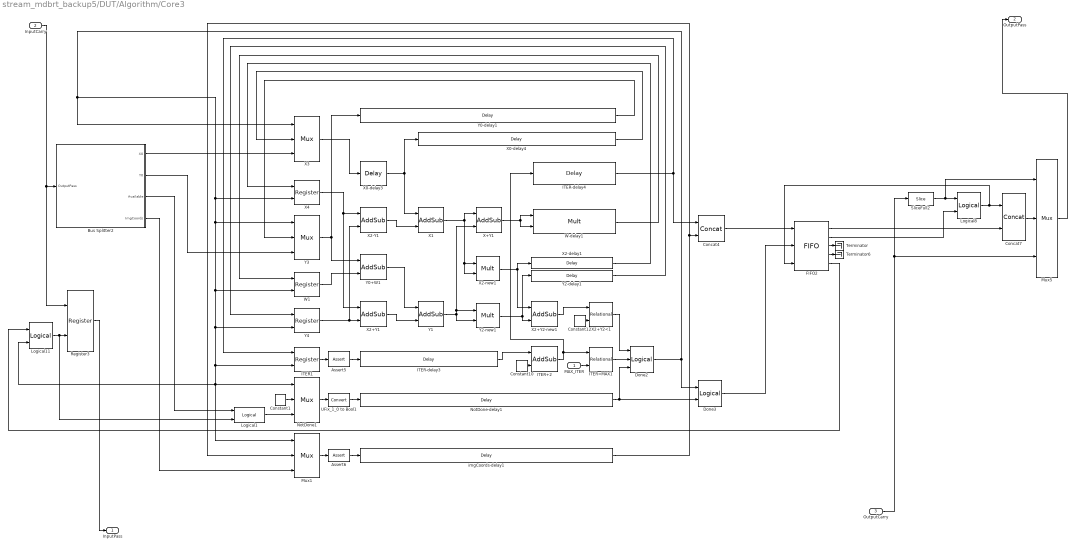
== system stream_mdbrt_backup5/DUT/Algorithm/Core3 ==
  MAX_ITER : Inport
  InputCarry : Inport  Port=2
  OutputCarry : Inport  Port=3
  Assert5 : hdlBasic/Assert  assert_type=on  type_source=Explicitly  gui_display_data_type=Fixed-point  arith_type=Unsigned  n_bits=bitsiter  bin_pt=0  preci_type=Single  exp_width=8  frac_width=24  assert_rate=off  rate_source=Explicitly  period=1  output_port=on  XmcBlockStatus=1  maskContainerNames=group1  block_type=assert  block_config=sysgen:assert_config  block_width=609  block_height=900
  Assert6 : hdlBasic/Assert  assert_type=on  type_source=Explicitly  gui_display_data_type=Fixed-point  arith_type=Unsigned  n_bits=bitswidth+bitsheight  bin_pt=0  preci_type=Single  exp_width=8  frac_width=24  assert_rate=off  rate_source=Explicitly  period=1  output_port=on  XmcBlockStatus=1  maskContainerNames=group1  block_type=assert  block_config=sysgen:assert_config  block_width=609  block_height=900
  Bus Splitter2 : Subsystem  TreatAsAtomicUnit=on
  Concat4 : hdlBasic/Concat  num_inputs=2  XmcBlockStatus=1  maskContainerNames=group1  block_type=concat  block_config=sysgen:Concat_config
  Concat7 : hdlBasic/Concat  num_inputs=2  XmcBlockStatus=1  maskContainerNames=group1  block_type=concat  block_config=sysgen:Concat_config
  Constant1 : hdlBasic/Constant  const=1  gui_display_data_type=Boolean  arith_type=Boolean  n_bits=bits  bin_pt=0  preci_type=Single  exp_width=8  frac_width=24  explicit_period=off  period=1  XmcBlockStatus=1  maskContainerNames=tabcontainer1  block_type=constant  block_config=sysgen:Constant_config
  Constant10 : hdlBasic/Constant  const=1  gui_display_data_type=Fixed-point  arith_type=Unsigned  n_bits=bits  bin_pt=0  preci_type=Single  exp_width=8  frac_width=24  explicit_period=off  period=1  XmcBlockStatus=1  maskContainerNames=tabcontainer1  block_type=constant  block_config=sysgen:Constant_config
  Constant12 : hdlBasic/Constant  const=4  gui_display_data_type=Fixed-point  arith_type=Signed (2's comp)  n_bits=bits  bin_pt=binpoint  preci_type=Single  exp_width=8  frac_width=24  explicit_period=off  period=1  XmcBlockStatus=1  maskContainerNames=tabcontainer1  block_type=constant  block_config=sysgen:Constant_config
  Done2 : hdlBasic/Logical  logical_function=NAND  inputs=3  en=off  latency=0  precision=User Defined  arith_type=Boolean  n_bits=1  bin_pt=0  align_bp=on  overflow=[]  quantization=[]  XmcBlockStatus=1  maskContainerNames=tabcontainer1  block_type=logical  block_config=sysgen:Logical_config
  Done3 : hdlBasic/Logical  logical_function=AND  inputs=2  en=off  latency=0  precision=User Defined  arith_type=Boolean  n_bits=1  bin_pt=0  align_bp=on  overflow=[]  quantization=[]  XmcBlockStatus=1  maskContainerNames=tabcontainer1  block_type=logical  block_config=sysgen:Logical_config
  FIFO2 : hdlBasic/FIFO  mem_type=Distributed RAM  performance_options=First_Word_Fall_Through  embedded_registers=off  depth=32  use_asym_data_widths=off  asym_read_width=32  percent_nbits=1  rst=off  rst_latency=1  en=off  use_dcount=off  use_percent_full_port=on  use_almost_empty=on  almost_empty_thresh=15  use_almost_full=off  use_rd_rst_busy=off  use_wr_rst_busy=off  almost_full_thresh=7  almost_empty_offset=[]  almost_full_offset=[]  explicit_period=off  period=[]  store_only_valid=[]  init_zero=[]  simulation_type=fast_sim  XmcBlockStatus=1  maskContainerNames=tabcontainer1  block_type=fifo  block_config=sysgen:FIFO_config  block_width=538  block_height=997
      settings: infoedit=[]
  ITER+2 : hdlBasic/AddSub  mode=Addition  use_carryin=off  use_carryout=off  en=off  latency=3  precision=User Defined  arith_type=Unsigned  n_bits=bitsiter  bin_pt=0  quantization=Truncate  overflow=Wrap  use_behavioral_HDL=off  hw_selection=Fabric  pipelined=off  XmcBlockStatus=1  maskContainerNames=tabcontainer1  block_type=addsub  block_config=sysgen:Addsub_config
  ITER-delay3 : hdlBasic/Delay  rst=off  en=off  latency=8  reg_retiming=off  XmcBlockStatus=1  maskContainerNames=group1  block_type=delay  block_config=sysgen:Delay_config
  ITER-delay4 : hdlBasic/Delay  rst=off  en=off  latency=2  reg_retiming=off  XmcBlockStatus=1  maskContainerNames=group1  block_type=delay  block_config=sysgen:Delay_config
  ITER1 : hdlBasic/Register  init=0  rst=on  en=off  XmcBlockStatus=1  maskContainerNames=tabcontainer1  block_type=register  block_config=sysgen:Register_config
  ITER<MAX1 : hdlBasic/Relational  mode=a<b  op_type=Bool  en=off  latency=2  XmcBlockStatus=1  maskContainerNames=tabcontainer1  block_type=relational  block_config=sysgen:Relational_config
  Logical1 : hdlBasic/Logical  logical_function=AND  inputs=2  en=off  latency=0  precision=Full  arith_type=Unsigned  n_bits=16  bin_pt=0  align_bp=on  overflow=[]  quantization=[]  XmcBlockStatus=1  maskContainerNames=tabcontainer1  block_type=logical  block_config=sysgen:Logical_config
  Logical11 : hdlBasic/Logical  logical_function=AND  inputs=2  en=off  latency=0  precision=Full  arith_type=Unsigned  n_bits=16  bin_pt=0  align_bp=on  overflow=[]  quantization=[]  XmcBlockStatus=1  maskContainerNames=tabcontainer1  block_type=logical  block_config=sysgen:Logical_config
  Logical8 : hdlBasic/Logical  logical_function=NOR  inputs=2  en=off  latency=0  precision=Full  arith_type=Unsigned  n_bits=16  bin_pt=0  align_bp=on  overflow=[]  quantization=[]  XmcBlockStatus=1  maskContainerNames=tabcontainer1  block_type=logical  block_config=sysgen:Logical_config
  Mux1 : hdlBasic/Mux  inputs=2  en=off  latency=1  precision=User Defined  arith_type=Unsigned  n_bits=bitswidth+bitsheight  bin_pt=0  quantization=Truncate  overflow=Wrap  XmcBlockStatus=1  maskContainerNames=tabcontainer1  block_type=mux  block_config=sysgen:Mux_config
  Mux5 : hdlBasic/Mux  inputs=2  en=off  latency=1  precision=User Defined  arith_type=Unsigned  n_bits=bitswidth+bitsheight+bitsiter+1  bin_pt=0  quantization=Truncate  overflow=Wrap  XmcBlockStatus=1  maskContainerNames=tabcontainer1  block_type=mux  block_config=sysgen:Mux_config
  NotDone-delay1 : hdlBasic/Delay  rst=off  en=off  latency=13  reg_retiming=off  XmcBlockStatus=1  maskContainerNames=group1  block_type=delay  block_config=sysgen:Delay_config
  NotDone1 : hdlBasic/Mux  inputs=2  en=off  latency=1  precision=User Defined  arith_type=Unsigned  n_bits=1  bin_pt=0  quantization=Truncate  overflow=Wrap  XmcBlockStatus=1  maskContainerNames=tabcontainer1  block_type=mux  block_config=sysgen:Mux_config
  Register3 : hdlBasic/Register  init=0  rst=on  en=off  XmcBlockStatus=1  maskContainerNames=tabcontainer1  block_type=register  block_config=sysgen:Register_config
  SliceFull2 : hdlBasic/Slice  nbits=1  boolean_output=on  mode=Upper Bit Location + Width  bit1=0  base1=MSB of Input  bit0=0  base0=LSB of Input  XmcBlockStatus=1  maskContainerNames=group1  block_type=slice  block_config=sysgen:Slice_config
  Terminator : Terminator
  Terminator6 : Terminator
  UFix_1_0 to Bool1 : hdlBasic/Convert  gui_display_data_type=Boolean  arith_type=Boolean  n_bits=16  bin_pt=14  float_type=Single  exp_bits=8  fraction_bits=24  quantization=Truncate  overflow=Wrap  en=off  latency=0  pipeline=off  XmcBlockStatus=1  maskContainerNames=group2  block_type=convert  block_config=sysgen:Convert_config  block_width=595  block_height=885
  W-delay1 : hdlBasic/Mult  precision=Full  arith_type="Signed  (2's comp)"  n_bits=16  bin_pt=14  quantization=Truncate  overflow=Wrap  en=off  latency=7  use_behavioral_HDL=off  opt=Speed  use_embedded=on  optimum_pipeline=off  pipeline=on  use_rpm=on  placement_style=Triangular  XmcBlockStatus=1  maskContainerNames=group1  block_type=mult  block_config=sysgen:Mult_config  block_width=598  block_height=876
  W1 : hdlBasic/Register  init=0  rst=on  en=off  XmcBlockStatus=1  maskContainerNames=tabcontainer1  block_type=register  block_config=sysgen:Register_config
  X+Y1 : hdlBasic/AddSub  mode=Addition  use_carryin=off  use_carryout=off  en=off  latency=4  precision=User Defined  arith_type="Signed  (2's comp)"  n_bits=bits  bin_pt=binpoint  quantization=Truncate  overflow=Wrap  use_behavioral_HDL=off  hw_selection=Fabric  pipelined=off  XmcBlockStatus=1  maskContainerNames=tabcontainer1  block_type=addsub  block_config=sysgen:Addsub_config
  X0-delay3 : hdlBasic/Delay  rst=off  en=off  latency=1  reg_retiming=off  XmcBlockStatus=1  maskContainerNames=group1  block_type=delay  block_config=sysgen:Delay_config
  X0-delay4 : hdlBasic/Delay  rst=off  en=off  latency=12  reg_retiming=off  XmcBlockStatus=1  maskContainerNames=group1  block_type=delay  block_config=sysgen:Delay_config
  X1 : hdlBasic/AddSub  mode=Addition  use_carryin=off  use_carryout=off  en=off  latency=1  precision=User Defined  arith_type="Signed  (2's comp)"  n_bits=bits  bin_pt=binpoint  quantization=Truncate  overflow=Wrap  use_behavioral_HDL=off  hw_selection=Fabric  pipelined=off  XmcBlockStatus=1  maskContainerNames=tabcontainer1  block_type=addsub  block_config=sysgen:Addsub_config
  X2+Y1 : hdlBasic/AddSub  mode=Addition  use_carryin=off  use_carryout=off  en=off  latency=1  precision=User Defined  arith_type="Signed  (2's comp)"  n_bits=bits  bin_pt=binpoint  quantization=Truncate  overflow=Wrap  use_behavioral_HDL=off  hw_selection=Fabric  pipelined=off  XmcBlockStatus=1  maskContainerNames=tabcontainer1  block_type=addsub  block_config=sysgen:Addsub_config
  X2+Y2-new1 : hdlBasic/AddSub  mode=Addition  use_carryin=off  use_carryout=off  en=off  latency=3  precision=User Defined  arith_type="Signed  (2's comp)"  n_bits=bits  bin_pt=binpoint  quantization=Truncate  overflow=Wrap  use_behavioral_HDL=off  hw_selection=Fabric  pipelined=off  XmcBlockStatus=1  maskContainerNames=tabcontainer1  block_type=addsub  block_config=sysgen:Addsub_config
  X2+Y2<1 : hdlBasic/Relational  mode=a<b  op_type=Bool  en=off  latency=2  XmcBlockStatus=1  maskContainerNames=tabcontainer1  block_type=relational  block_config=sysgen:Relational_config
  X2-Y1 : hdlBasic/AddSub  mode=Subtraction  use_carryin=off  use_carryout=off  en=off  latency=1  precision=User Defined  arith_type="Signed  (2's comp)"  n_bits=bits  bin_pt=binpoint  quantization=Truncate  overflow=Wrap  use_behavioral_HDL=off  hw_selection=Fabric  pipelined=off  XmcBlockStatus=1  maskContainerNames=tabcontainer1  block_type=addsub  block_config=sysgen:Addsub_config
  X2-delay1 : hdlBasic/Delay  rst=off  en=off  latency=5  reg_retiming=off  XmcBlockStatus=1  maskContainerNames=group1  block_type=delay  block_config=sysgen:Delay_config
  X2-new1 : hdlBasic/Mult  precision=Full  arith_type="Signed  (2's comp)"  n_bits=16  bin_pt=14  quantization=Truncate  overflow=Wrap  en=off  latency=6  use_behavioral_HDL=off  opt=Speed  use_embedded=on  optimum_pipeline=off  pipeline=on  use_rpm=on  placement_style=Triangular  XmcBlockStatus=1  maskContainerNames=group1  block_type=mult  block_config=sysgen:Mult_config  block_width=598  block_height=876
  X3 : hdlBasic/Mux  inputs=2  en=off  latency=1  precision=User Defined  arith_type="Signed  (2's comp)"  n_bits=bits  bin_pt=binpoint  quantization=Truncate  overflow=Wrap  XmcBlockStatus=1  maskContainerNames=tabcontainer1  block_type=mux  block_config=sysgen:Mux_config
  X4 : hdlBasic/Register  init=0  rst=on  en=off  XmcBlockStatus=1  maskContainerNames=tabcontainer1  block_type=register  block_config=sysgen:Register_config
  Y0+W1 : hdlBasic/AddSub  mode=Addition  use_carryin=off  use_carryout=off  en=off  latency=1  precision=User Defined  arith_type="Signed  (2's comp)"  n_bits=bits  bin_pt=binpoint  quantization=Truncate  overflow=Wrap  use_behavioral_HDL=off  hw_selection=Fabric  pipelined=off  XmcBlockStatus=1  maskContainerNames=tabcontainer1  block_type=addsub  block_config=sysgen:Addsub_config
  Y0-delay1 : hdlBasic/Delay  rst=off  en=off  latency=13  reg_retiming=off  XmcBlockStatus=1  maskContainerNames=group1  block_type=delay  block_config=sysgen:Delay_config
  Y1 : hdlBasic/AddSub  mode=Subtraction  use_carryin=off  use_carryout=off  en=off  latency=1  precision=User Defined  arith_type="Signed  (2's comp)"  n_bits=bits  bin_pt=binpoint  quantization=Truncate  overflow=Wrap  use_behavioral_HDL=off  hw_selection=Fabric  pipelined=off  XmcBlockStatus=1  maskContainerNames=tabcontainer1  block_type=addsub  block_config=sysgen:Addsub_config
  Y2-delay1 : hdlBasic/Delay  rst=off  en=off  latency=5  reg_retiming=off  XmcBlockStatus=1  maskContainerNames=group1  block_type=delay  block_config=sysgen:Delay_config
  Y2-new1 : hdlBasic/Mult  precision=Full  arith_type="Signed  (2's comp)"  n_bits=16  bin_pt=14  quantization=Truncate  overflow=Wrap  en=off  latency=6  use_behavioral_HDL=off  opt=Speed  use_embedded=on  optimum_pipeline=off  pipeline=on  use_rpm=on  placement_style=Triangular  XmcBlockStatus=1  maskContainerNames=group1  block_type=mult  block_config=sysgen:Mult_config  block_width=598  block_height=876
  Y3 : hdlBasic/Mux  inputs=2  en=off  latency=1  precision=User Defined  arith_type="Signed  (2's comp)"  n_bits=bits  bin_pt=binpoint  quantization=Truncate  overflow=Wrap  XmcBlockStatus=1  maskContainerNames=tabcontainer1  block_type=mux  block_config=sysgen:Mux_config
  Y4 : hdlBasic/Register  init=0  rst=on  en=off  XmcBlockStatus=1  maskContainerNames=tabcontainer1  block_type=register  block_config=sysgen:Register_config
  imgCoords-delay1 : hdlBasic/Delay  rst=off  en=off  latency=13  reg_retiming=off  XmcBlockStatus=1  maskContainerNames=group1  block_type=delay  block_config=sysgen:Delay_config
  InputPass : Outport
  OutputPass : Outport  Port=2
  wires:
  NotDone1/1 -> UFix_1_0 to Bool1/1
  SliceFull2/1 -> Mux5/1, Logical8/1
  ITER-delay3/1 -> ITER+2/1
  Y4/1 -> X2-Y1/2, X2+Y1/2
  Y2-delay1/1 -> Y4/1
  Done3/1 -> FIFO2/2
  Assert6/1 -> imgCoords-delay1/1
  InputCarry/1 -> Register3/1, Bus Splitter2/1(OutputPass)
  X1/1 -> X2-new1/2, X2-new1/1, X+Y1/1
  X2-delay1/1 -> X4/1
  Done2/1 -> Done3/1, X4/2, Y3/1, W1/2, ITER1/2, Logical11/2, Mux1/1, NotDone1/1, Y4/2, X3/1
  W1/1 -> Y0+W1/2
  Constant10/1 -> ITER+2/2
  Logical8/1 -> FIFO2/3, Concat7/1
  FIFO2/2 -> Logical8/2
  X2+Y2-new1/1 -> X2+Y2<1/1
  Bus Splitter2/1(X0) -> X3/3
  X2+Y1/1 -> Y1/2
  Logical11/1 -> Logical1/2, Register3/2
  NotDone-delay1/1 -> Done2/3, Done3/2
  OutputCarry/1 -> SliceFull2/1, Mux5/3
  Mux5/1 -> OutputPass/1
  FIFO2/3 -> Terminator/1
  ITER-delay4/1 -> Concat4/1, ITER1/1
  Y3/1 -> Y0+W1/1, Y0-delay1/1
  Register3/1 -> InputPass/1
  X4/1 -> X2+Y1/1, X2-Y1/1
  ITER+2/1 -> ITER-delay4/1, ITER<MAX1/1
  Y1/1 -> X+Y1/2, Y2-new1/1, Y2-new1/2
  Y2-new1/1 -> Y2-delay1/1, X2+Y2-new1/2
  ITER<MAX1/1 -> Done2/2
  Constant12/1 -> X2+Y2<1/2
  Y0+W1/1 -> Y1/1
  Assert5/1 -> ITER-delay3/1
  UFix_1_0 to Bool1/1 -> NotDone-delay1/1
  X2+Y2<1/1 -> Done2/1
  imgCoords-delay1/1 -> Mux1/2, Concat4/2
  FIFO2/5 -> Logical11/1
  Bus Splitter2/4(ImgCoords) -> Mux1/3
  X2-Y1/1 -> X1/2
  ITER1/1 -> Assert5/1
  X+Y1/1 -> W-delay1/2, W-delay1/1
  X0-delay3/1 -> X0-delay4/1, X1/1
  Y0-delay1/1 -> Y3/2
  X3/1 -> X0-delay3/1
  Concat7/1 -> Mux5/2
  X0-delay4/1 -> X3/2
  X2-new1/1 -> X2-delay1/1, X2+Y2-new1/1
  Bus Splitter2/2(Y0) -> Y3/3
  W-delay1/1 -> W1/1
  MAX_ITER/1 -> ITER<MAX1/2
  Bus Splitter2/3(Available) -> Logical1/1
  FIFO2/4 -> Terminator6/1
  Mux1/1 -> Assert6/1
  Concat4/1 -> FIFO2/1
  FIFO2/1 -> Concat7/2
  Constant1/1 -> NotDone1/2
  Logical1/1 -> NotDone1/3
